simulink model "simulation_2021b"  (R2021b)
settings: Solver=FixedStepAuto  StartTime=0.0  StopTime=T  RelTol=1e-3  EnableMultiTasking=on
undefined symbols (not defined in the file or in its folder): disc, discrete_0, h, K, Ts
libraries: eeLuenbergerObserver x1, simulink x1
settings Model: Creator=rbabuska  LastModifiedBy=wilbe
settings SolverCC: AlgebraicLoopSolver=TrustRegion  AutoInsertRateTranBlk=on
settings DataIOCC: LimitDataPoints=on  SaveFormat=Array  SignalLoggingSaveFormat=ModelDataLogs  SaveOutput=off  SaveTime=off  ReturnWorkspaceOutputs=off
settings OptimizationCC: DefaultParameterBehavior=Inlined  InlineInvariantSignals=on  EnhancedBackFolding=on  PassReuseOutputArgsAs=Individual arguments  ExpressionDepthLimit=2147483647  StateBitsets=on  DataBitsets=on  ZeroExternalMemoryAtStartup=off  ZeroInternalMemoryAtStartup=off  NoFixptDivByZeroProtection=on  LifeSpan=1  OptimizeBlockOrder=speed  DifferentSizesBufferReuse=on  EfficientTunableParamExpr=on
settings DebuggingCC: UnderspecifiedInitializationDetection=Classic  MergeDetectMultiDrivingBlocksExec=none  ParameterTunabilityLossMsg=error  FcnCallInpInsideContextMsg=warning  StateNameClashWarn=warning  SFUnexpectedBacktrackingDiag=warning  SFNoUnconditionalDefaultTransitionDiag=warning  SFExecutionAtInitializationDiag=none  SFMachineParentedDataDiag=warning  ArithmeticOperatorsInVariantConditions=warning
settings HardwareCC: ProdBitPerPointer=32  ProdBitPerSizeT=32  ProdBitPerPtrDiffT=32  ProdLargestAtomicFloat=None  ProdIntDivRoundTo=Floor  ProdWordSize=32  ProdHWDeviceType=Generic->Custom
settings ModelReferenceCC: PropagateSignalLabelsOutOfModel=off
settings SFSimCC: SimUseLocalCustomCode=off  MATLABDynamicMemAlloc=off  CustomCodeUndefinedFunction=UseInterfaceOnly
settings RTWCC: Description=Embedded Coder  SystemTargetFile=ert.tlc  TLCOptions=-p0  GenCodeOnly=on  TemplateMakefile=ert_default_tmf  GenerateReport=on  RTWVerbose=off  RTWUseLocalCustomCode=off  IncludeHyperlinkInReport=on  LaunchReport=on
settings CodeAppCC: ForceParamTrailComments=on  IgnoreCustomStorageClasses=off  OperatorAnnotations=on  SimulinkDataObjDesc=on  SFDataObjDesc=on  CustomSymbolStrGlobalVar=rt$N$M  CustomSymbolStrType=$N$M  CustomSymbolStrFcn=$N$M$F  CustomSymbolStrMacro=$N$M  InsertBlockDesc=on
settings ERTTargetCC: CodeReplacementLibrary=ISO_C  GenerateSampleERTMain=on  IncludeMdlTerminateFcn=off  SuppressErrorStatus=on  SupportAbsoluteTime=off  PurelyIntegerCode=on  SupportNonFinite=off  SupportComplex=off  InlinedParameterPlacement=NonHierarchical  RootIOFormat=Structure reference  ERTCustomFileTemplate=example_file_process.tlc
settings ConfigComp: CovMetricSettings=dw  CovSaveCumulativeToWorkspaceVar=on  CovSaveSingleToWorkspaceVar=on  CovExternalEMLEnable=off  CovSFcnEnable=off

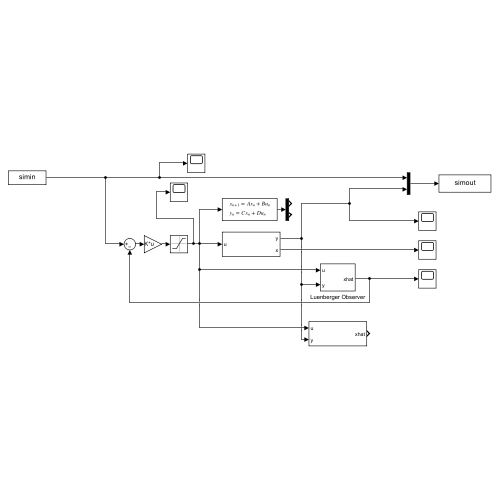
[thumbnail: Simulink's stored preview of the top-level diagram]
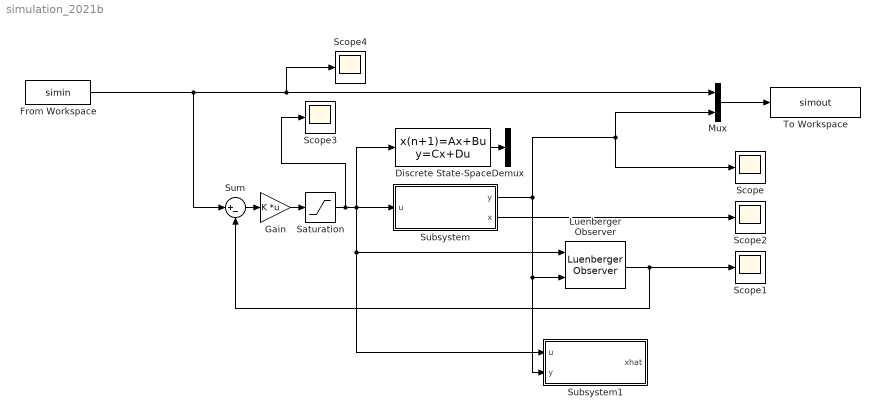
== system simulation_2021b ==
  Demux : Demux  Outputs=[2;4]
  Discrete State-Space : DiscreteStateSpace  A=discrete_0.A  B=discrete_0.B  C=[discrete_0.C;eye(4)]  D=[discrete_0.D;zeros(4,1)]  InitialCondition=[0;0;0;0]  SampleTime=h
  From Workspace : FromWorkspace  VariableName=simin  SampleTime=h  OutputAfterFinalValue=Holding final value
  Gain : Gain  Gain=K  Multiplication=Matrix(K*u)
  Luenberger Observer : eeLuenbergerObserver/Luenberger Observer  StateSpaceType=Discrete-time  Ad=discrete_0.A  Bd=discrete_0.B  Cd=discrete_0.C  Dd=discrete_0.D  A=1  B=1  C=1  D=1  ObserverDesign=Desired eigenvalues  Ld=[1,1]  DesiredEigenvalues=pDisc  x0=[0;0;0;0]  Tsd=0.1  Ts=h
  Mux : Mux  Inputs=2
  Saturation : Saturate  UpperLimit=0.08  LowerLimit=-0.08
  Scope{,1..4} (5 alike) : Scope
  Subsystem : Subsystem
  Subsystem1 : Subsystem
  Sum : Sum  Inputs=|+-
  To Workspace : ToWorkspace  VariableName=simout  SaveFormat=Timeseries  SampleTime=-1
  wires:
  From Workspace/1 -> Scope4/1, Mux/1, Sum/1
  Mux/1 -> To Workspace/1
  Subsystem/1(y) -> Scope/1, Mux/2, Subsystem1/2(y), Luenberger Observer/2
  Luenberger Observer/1 -> Scope1/1, Sum/2
  Discrete State-Space/1 -> Demux/1
  Subsystem/2(x) -> Scope2/1
  Sum/1 -> Gain/1
  Gain/1 -> Saturation/1
  Saturation/1 -> Scope3/1, Subsystem1/1(u), Luenberger Observer/1, Discrete State-Space/1, Subsystem/1(u)

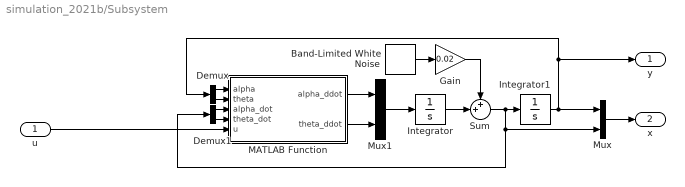
== system simulation_2021b/Subsystem ==
  u : Inport
  Band-Limited White Noise : simulink/Sources/Band-Limited White Noise  Cov=[0.02]  Ts=0.1  seed=[23341]
  Demux : Demux  Outputs=2
  Demux1 : Demux  Outputs=2
  Gain : Gain  Gain=0.02
  Integrator : Integrator
  Integrator1 : Integrator
  MATLAB Function : MATLAB Function  TreatAsAtomicUnit=on
  Mux : Mux  Inputs=2
  Mux1 : Mux  Inputs=2
  Sum : Sum  Inputs=++|
  y : Outport  PortDimensions=2
  x : Outport  Port=2  PortDimensions=4
  wires:
  Integrator/1 -> Sum/2
  Sum/1 -> Mux/2, Demux1/1, Integrator1/1
  MATLAB Function/2(theta_ddot) -> Mux1/2
  MATLAB Function/1(alpha_ddot) -> Mux1/1
  Demux/2 -> MATLAB Function/2(theta)
  Demux/1 -> MATLAB Function/1(alpha)
  Integrator1/1 -> Demux/1, y/1, Mux/1
  Mux1/1 -> Integrator/1
  Demux1/2 -> MATLAB Function/4(theta_dot)
  Demux1/1 -> MATLAB Function/3(alpha_dot)
  u/1 -> MATLAB Function/5(u)
  Band-Limited White Noise/1 -> Gain/1
  Gain/1 -> Sum/1
  Mux/1 -> x/1

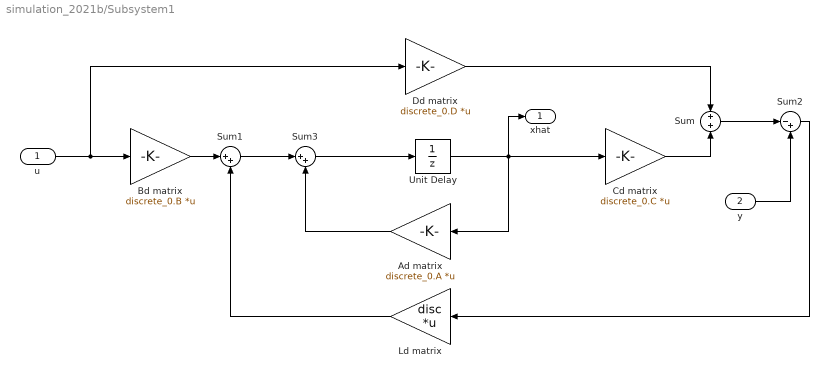
== system simulation_2021b/Subsystem1 ==
  u : Inport  SampleTime=Ts
  y : Inport  Port=2  SampleTime=Ts
  Ad matrix : Gain  Gain=discrete_0.A  Multiplication=Matrix(K*u)
  Bd matrix : Gain  Gain=discrete_0.B  Multiplication=Matrix(K*u)
  Cd matrix : Gain  Gain=discrete_0.C  Multiplication=Matrix(K*u)
  Dd matrix : Gain  Gain=discrete_0.D  Multiplication=Matrix(K*u)
  Ld matrix : Gain  Gain=disc  Multiplication=Matrix(K*u)
  Sum : Sum
  Sum1 : Sum  Inputs=|++
  Sum2 : Sum  Inputs=|-+
  Sum3 : Sum  Inputs=|++
  Unit Delay : UnitDelay  InitialCondition=[0;0;0;0]'  SampleTime=Ts  HasFrameUpgradeWarning=on
  xhat : Outport  VectorParamsAs1DForOutWhenUnconnected=off
  wires:
  Dd matrix/1 -> Sum/1
  Sum3/1 -> Unit Delay/1
  y/1 -> Sum2/2
  Ld matrix/1 -> Sum1/2
  Unit Delay/1 -> Ad matrix/1, xhat/1, Cd matrix/1
  Sum/1 -> Sum2/1
  Cd matrix/1 -> Sum/2
  Sum1/1 -> Sum3/1
  u/1 -> Bd matrix/1, Dd matrix/1
  Ad matrix/1 -> Sum3/2
  Bd matrix/1 -> Sum1/1
  Sum2/1 -> Ld matrix/1

== matlab function simulation_2021b/Subsystem/MATLAB Function ==
  data: alpha input; theta input; alpha_dot input; theta_dot input; alpha_ddot output; u input; theta_ddot output
function [alpha_ddot,theta_ddot] = fcn(alpha,theta,alpha_dot,theta_dot,u)
alpha_ddot=((alpha_dot.*(-2.46872604672e-5)+u.*1.9980288e-3+theta_dot.^2.*sin(theta).*9.47552256e-7+cos(theta).*sin(theta).*4.5993298176e-4+theta_dot.*cos(theta).*8.22528e-7).*(-5.0./8.4e+1))./(cos(theta).^2.*5.992704e-8-1.4533632e-7);
theta_ddot=((theta_dot.*1.059744e-6+sin(theta).*5.9257705248e-4-alpha_dot.*cos(theta).*1.31151071232e-5+u.*cos(theta).*1.0614528e-3+theta_dot.^2.*cos(theta).*sin(theta).*5.03387136e-7).*(5.0./4.2e+1))./(cos(theta).^2.*5.992704e-8-1.4533632e-7);
